simulink model "control_cdr_hybrid"  (Simulink 7.8)
settings: Solver=ode5  StartTime=0.0  StopTime=100  FixedStep=0.001  RelTol=1e-3
undefined symbols (not defined in the file): DamperOFF, DiscIntNeverNeededParam, Ki_L1, Ki_R1, Ki_R3, Kp_L1, Kp_R1, Kp_R2, Kp_R3, Matlab_version, Output_File, Output_file_n, Plant_inputs_num, Plant_outputs_num, polys, RecurDyn, RecurDyn_controltimestep, RecurDyn_model, RecurDyn_model_n, sigbuilder_block, SpringOFF, StaticTorque_RW1, StaticTorque_RW2, Ts, Tuning, Wheel_Vel
(part 1 of 2)
settings Model: Creator=sonyi  LastModifiedBy=ecsl
settings OptimizationCC: InitFltsAndDblsToZero=on
settings DebuggingCC: FcnCallInpInsideContextMsg=Use local settings  StrictBusMsg=Warning
settings SimEventsCC: propDiagStatOutput=1

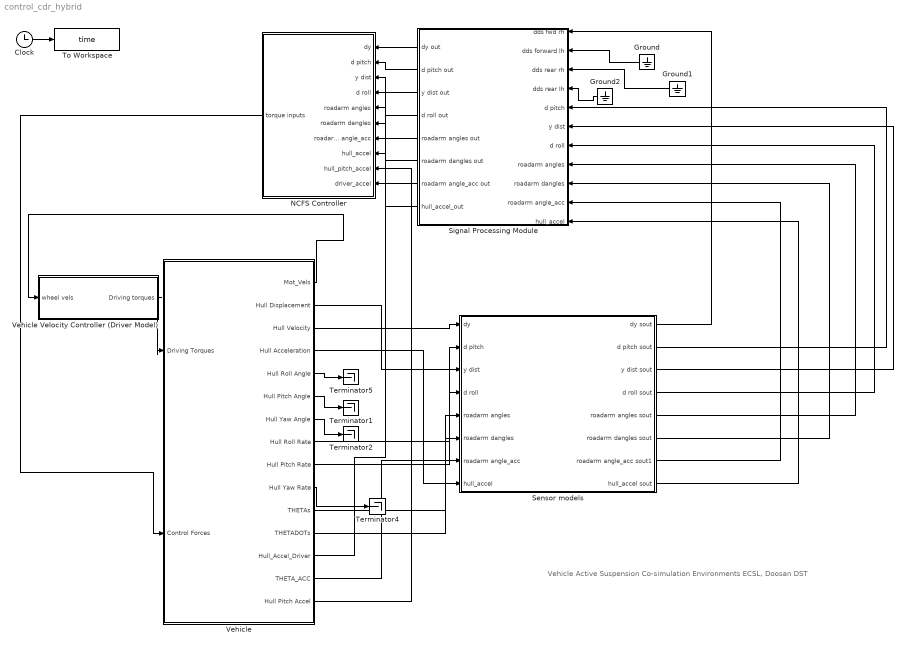
== system control_cdr_hybrid ==
  note: Vehicle Active Suspension Co-simulation Environments
      | ECSL, Doosan DST
  Clock : Clock
  Ground : Ground
  Ground1 : Ground
  Ground2 : Ground
  NCFS Controller : Subsystem
  Sensor models : Subsystem
  Signal Processing Module : Subsystem
  Terminator{1..2,4..5} (4 alike) : Terminator
  To Workspace : ToWorkspace  VariableName=time  SampleTime=-1  SaveFormat=Array
  Vehicle : Subsystem
  Vehicle Velocity Controller (Driver Model) : Subsystem
  wires:
  Vehicle/1(Mot_Vels) -> Vehicle Velocity Controller (Driver Model)/1(wheel vels)
  Clock/1 -> To Workspace/1
  Signal Processing Module/1(dy out) -> NCFS Controller/1(dy)
  Signal Processing Module/3(y dist out) -> NCFS Controller/3(y dist)
  Signal Processing Module/2(d pitch out) -> NCFS Controller/2(d pitch)
  Signal Processing Module/5(roadarm angles out) -> NCFS Controller/5(roadarm angles)
  Signal Processing Module/4(d roll out) -> NCFS Controller/4(d roll)
  Signal Processing Module/6(roadarm dangles out) -> NCFS Controller/6(roadarm dangles)
  Sensor models/1(dy sout) -> Signal Processing Module/1(dds fwd rh)
  Sensor models/2(d pitch sout) -> Signal Processing Module/5(d pitch)
  Sensor models/3(y dist sout) -> Signal Processing Module/6(y dist)
  Sensor models/4(d roll sout) -> Signal Processing Module/7(d roll)
  Sensor models/5(roadarm angles sout) -> Signal Processing Module/8(roadarm angles)
  Sensor models/6(roadarm dangles sout) -> Signal Processing Module/9(roadarm dangles)
  NCFS Controller/1(torque inputs) -> Vehicle/2(Control Forces)
  Sensor models/7(roadarm angle_acc sout1) -> Signal Processing Module/10(roadarm angle_acc)
  Signal Processing Module/7(roadarm angle_acc out) -> NCFS Controller/7(roadarm angle_acc)
  Sensor models/8(hull_accel sout) -> Signal Processing Module/11(hull_accel)
  Signal Processing Module/8(hull_accel_out) -> NCFS Controller/8(hull_accel)
  Ground/1 -> Signal Processing Module/2(dds forward lh)
  Ground1/1 -> Signal Processing Module/3(dds rear rh)
  Ground2/1 -> Signal Processing Module/4(dds rear lh)
  Vehicle/2(Hull Displacement) -> Sensor models/3(y dist)
  Vehicle/3(Hull Velocity) -> Sensor models/1(dy)
  Vehicle/4(Hull Acceleration) -> Sensor models/8(hull_accel)
  Vehicle/8(Hull Roll Rate) -> Sensor models/4(d roll)
  Vehicle/11(THETAs) -> Sensor models/5(roadarm angles)
  Vehicle/12(THETADOTs) -> Sensor models/6(roadarm dangles)
  Vehicle/5(Hull Roll Angle) -> Terminator5/1
  Vehicle/6(Hull Pitch Angle) -> Terminator1/1
  Vehicle/7(Hull Yaw Angle) -> Terminator2/1
  Vehicle/9(Hull Pitch Rate) -> Sensor models/2(d pitch)
  Vehicle/10(Hull Yaw Rate) -> Terminator4/1
  Vehicle/14(THETA_ACC) -> Sensor models/7(roadarm angle_acc)
  Vehicle Velocity Controller (Driver Model)/1(Driving torques) -> Vehicle/1(Driving Torques)
  Vehicle/15(Hull Pitch Accel) -> NCFS Controller/9(hull_pitch_accel)
  Vehicle/13(Hull_Accel_Driver) -> NCFS Controller/10(driver_accel)

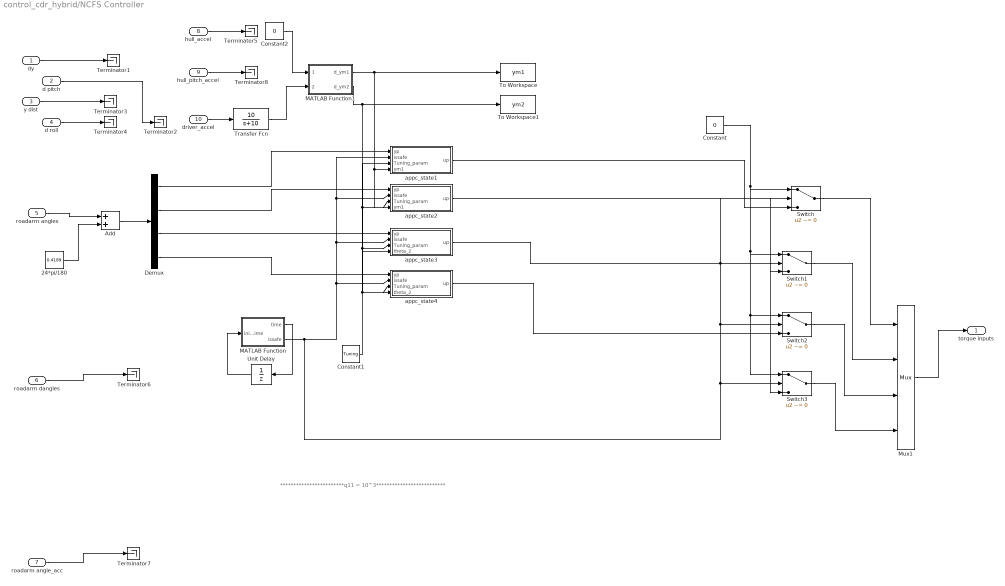
== system control_cdr_hybrid/NCFS Controller ==
  note: ************************q11 = 10^3**************************
  dy : Inport
  d pitch : Inport  Port=2
  y dist : Inport  Port=3
  d roll : Inport  Port=4
  roadarm angles : Inport  Port=5
  roadarm dangles : Inport  Port=6
  roadarm angle_acc : Inport  Port=7
  hull_accel : Inport  Port=8
  hull_pitch_accel : Inport  Port=9
  driver_accel : Inport  Port=10
  24*pi/180 : Constant  Value=0.4189
  Add : Sum
  Constant : Constant  Value=0
  Constant1 : Constant  Value=Tuning
  Constant2 : Constant  Value=0
  Demux : Demux
  MATLAB Function : MATLAB Function  TreatAsAtomicUnit=on
  MATLAB Function1 : MATLAB Function  TreatAsAtomicUnit=on
  Mux1 : Mux
  Switch{,1..3} (4 alike) : Switch  Criteria=u2 ~= 0
  Terminator{1..8} (8 alike) : Terminator
  To Workspace : ToWorkspace  VariableName=ym1  SampleTime=-1  SaveFormat=Array
  To Workspace1 : ToWorkspace  VariableName=ym2  SampleTime=-1  SaveFormat=Array
  Transfer Fcn : TransferFcn  Numerator=[10]  Denominator=[1 10]
  Unit Delay : UnitDelay  X0=3000  SampleTime=-1
  appc_state1 : Subsystem
  appc_state2 : Subsystem
  appc_state3 : Subsystem
  appc_state4 : Subsystem
  torque inputs : Outport
  wires:
  dy/1 -> Terminator1/1
  y dist/1 -> Terminator3/1
  d roll/1 -> Terminator4/1
  Mux1/1 -> torque inputs/1
  roadarm angles/1 -> Add/1
  24*pi/180/1 -> Add/2
  Add/1 -> Demux/1
  d pitch/1 -> Terminator2/1
  roadarm dangles/1 -> Terminator6/1
  roadarm angle_acc/1 -> Terminator7/1
  Demux/1 -> appc_state1/1(yp)
  Demux/2 -> appc_state2/1(yp)
  Demux/3 -> appc_state3/1(yp)
  Demux/4 -> appc_state4/1(yp)
  Constant1/1 -> appc_state1/3(Tuning_param), appc_state2/3(Tuning_param), appc_state3/3(Tuning_param), appc_state4/3(Tuning_param)
  appc_state3/1(up) -> Switch2/3
  appc_state4/1(up) -> Switch3/3
  appc_state1/1(up) -> Switch/3
  Constant/1 -> Switch/1, Switch3/1, Switch2/1, Switch1/1
  Unit Delay/1 -> MATLAB Function/1(init_time)
  MATLAB Function/1(time) -> Unit Delay/1
  MATLAB Function/2(issafe) -> appc_state4/2(issafe), appc_state3/2(issafe), appc_state2/2(issafe), appc_state1/2(issafe), Switch/2, Switch1/2, Switch2/2, Switch3/2
  appc_state2/1(up) -> Switch1/3
  MATLAB Function1/1(d_ym1) -> To Workspace/1, appc_state1/4(ym1), appc_state2/4(ym1)
  MATLAB Function1/2(d_ym2) -> To Workspace1/1, appc_state3/4(theta_2), appc_state4/4(theta_2)
  Switch/1 -> Mux1/1
  Switch1/1 -> Mux1/2
  Switch2/1 -> Mux1/3
  Switch3/1 -> Mux1/4
  Constant2/1 -> MATLAB Function1/1(pitch_acc)
  Transfer Fcn/1 -> MATLAB Function1/2(hull_acc)
  hull_pitch_accel/1 -> Terminator8/1
  hull_accel/1 -> Terminator5/1
  driver_accel/1 -> Transfer Fcn/1

== system control_cdr_hybrid/Sensor models ==
  dy : Inport
  d pitch : Inport  Port=2
  y dist : Inport  Port=3
  d roll : Inport  Port=4
  roadarm angles : Inport  Port=5
  roadarm dangles : Inport  Port=6
  roadarm angle_acc : Inport  Port=7
  hull_accel : Inport  Port=8
  dy sout : Outport
  d pitch sout : Outport  Port=2
  y dist sout : Outport  Port=3
  d roll sout : Outport  Port=4
  roadarm angles sout : Outport  Port=5
  roadarm dangles sout : Outport  Port=6
  roadarm angle_acc sout1 : Outport  Port=7
  hull_accel sout : Outport  Port=8
  wires:
  dy/1 -> dy sout/1
  y dist/1 -> y dist sout/1
  d pitch/1 -> d pitch sout/1
  roadarm angles/1 -> roadarm angles sout/1
  d roll/1 -> d roll sout/1
  roadarm dangles/1 -> roadarm dangles sout/1
  roadarm angle_acc/1 -> roadarm angle_acc sout1/1
  hull_accel/1 -> hull_accel sout/1

== system control_cdr_hybrid/Signal Processing Module ==
  dds fwd rh : Inport
  dds forward lh : Inport  Port=2
  dds rear rh : Inport  Port=3
  dds rear lh : Inport  Port=4
  d pitch : Inport  Port=5
  y dist : Inport  Port=6
  d roll : Inport  Port=7
  roadarm angles : Inport  Port=8
  roadarm dangles : Inport  Port=9
  roadarm angle_acc : Inport  Port=10
  hull_accel : Inport  Port=11
  Terminator : Terminator
  Terminator1 : Terminator
  Terminator2 : Terminator
  dy out : Outport
  d pitch out : Outport  Port=2
  y dist out : Outport  Port=3
  d roll out : Outport  Port=4
  roadarm angles out : Outport  Port=5
  roadarm dangles out : Outport  Port=6
  roadarm angle_acc out : Outport  Port=7
  hull_accel_out : Outport  Port=8
  wires:
  dds fwd rh/1 -> dy out/1
  y dist/1 -> y dist out/1
  d pitch/1 -> d pitch out/1
  roadarm angles/1 -> roadarm angles out/1
  d roll/1 -> d roll out/1
  roadarm dangles/1 -> roadarm dangles out/1
  roadarm angle_acc/1 -> roadarm angle_acc out/1
  hull_accel/1 -> hull_accel_out/1
  dds rear lh/1 -> Terminator2/1
  dds rear rh/1 -> Terminator1/1
  dds forward lh/1 -> Terminator/1

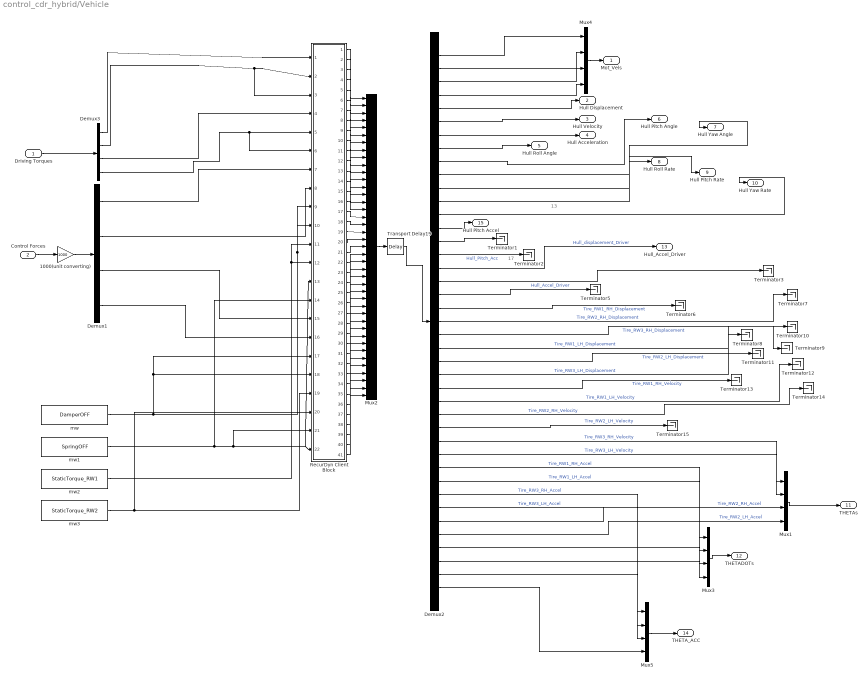
== system control_cdr_hybrid/Vehicle ==
  note: 13
  note: 17
  Driving Torques : Inport
  Control Forces : Inport  Port=2
  1000(unit converting) : Gain  Gain=1000
  Demux1 : Demux
  Demux2 : Demux  Outputs=41
  Demux3 : Demux
  Mux{1,3..5} (4 alike) : Mux
  Mux2 : Mux  Inputs=41
  RecurDyn Client Block : Subsystem
      mask Display: image(imread('basic_recurdyn2_client.TIF'))
  Terminator{1..3,5..15} (14 alike) : Terminator
  Transport Delay19 : TransportDelay  DelayTime=0.001
  mw : Constant  Value=DamperOFF
  mw1 : Constant  Value=SpringOFF
  mw2 : Constant  Value=StaticTorque_RW1
  mw3 : Constant  Value=StaticTorque_RW2
  Mot_Vels : Outport
  Hull Displacement : Outport  Port=2
  Hull Velocity : Outport  Port=3
  Hull Acceleration : Outport  Port=4
  Hull Roll Angle : Outport  Port=5
  Hull Pitch Angle : Outport  Port=6
  Hull Yaw Angle : Outport  Port=7
  Hull Roll Rate : Outport  Port=8
  Hull Pitch Rate : Outport  Port=9
  Hull Yaw Rate : Outport  Port=10
  THETAs : Outport  Port=11
  THETADOTs : Outport  Port=12
  Hull_Accel_Driver : Outport  Port=13
  THETA_ACC : Outport  Port=14
  Hull Pitch Accel : Outport  Port=15
  wires:
  Demux3/2 -> RecurDyn Client Block/2("Mot_Input_R2            "), RecurDyn Client Block/3("Mot_Input_R3            ")
  Demux3/1 -> RecurDyn Client Block/1("Mot_Input_R1            ")
  Transport Delay19/1 -> Demux2/1
  Mux2/1 -> Transport Delay19/1
  Driving Torques/1 -> Demux3/1
  Control Forces/1 -> 1000(unit converting)/1
  1000(unit converting)/1 -> Demux1/1
  Demux1/1 -> RecurDyn Client Block/7("Torque_RW1_RH@Arm1      ")
  Demux1/2 -> RecurDyn Client Block/8("Torque_RW1_LH@Arm1      ")
  mw/1 -> RecurDyn Client Block/9("DamperOFF_RW1_RH@Arm1   "), RecurDyn Client Block/10("DamperOFF_RW1_LH@Arm1   "), RecurDyn Client Block/17("DamperOFF_RW2_RH@Arm2   "), RecurDyn Client Block/18("DamperOFF_RW2_LH@Arm2   ")
  mw2/1 -> RecurDyn Client Block/11(StaticTorque_RW1_RH@Arm1), RecurDyn Client Block/12(StaticTorque_RW1_LH@Arm1)
  mw1/1 -> RecurDyn Client Block/13("SpringOFF_RW1_RH@Arm1   "), RecurDyn Client Block/21("SpringOFF_RW2_RH@Arm2   "), RecurDyn Client Block/22("SpringOFF_RW2_LH@Arm2   "), RecurDyn Client Block/14("SpringOFF_RW1_LH@Arm1   ")
  Demux1/3 -> RecurDyn Client Block/15("Torque_RW2_RH@Arm2      ")
  Demux1/4 -> RecurDyn Client Block/16("Torque_RW2_LH@Arm2      ")
  Mux4/1 -> Mot_Vels/1
  Demux2/1 -> Mux4/1
  Demux2/2 -> Mux4/2
  Demux2/3 -> Mux4/3
  Demux2/4 -> Mux4/4
  Demux2/5 -> Hull Displacement/1
  Demux2/6 -> Hull Velocity/1
  Demux2/7 -> Hull Acceleration/1
  Demux2/8 -> Hull Roll Angle/1
  Demux2/9 -> Hull Pitch Angle/1
  Demux2/10 -> Hull Yaw Angle/1
  Demux2/11 -> Hull Roll Rate/1
  Demux2/12 -> Hull Pitch Rate/1
  Demux2/13 -> Hull Yaw Rate/1
  Mux3/1 -> THETADOTs/1
  Mux1/1 -> THETAs/1
  Mux5/1 -> THETA_ACC/1
  Demux2/14 -> Hull Pitch Accel/1
  Demux2/15 -> Terminator1/1
  Demux2/16 -> Terminator2/1  "Hull_Pitch_Acc"
  Demux2/17 -> Hull_Accel_Driver/1  "Hull_displacement_Driver"
  Demux2/18 -> Terminator3/1
  Demux2/19 -> Terminator5/1  "Hull_Accel_Driver"
  Demux2/41 -> Mux5/4
  Demux2/40 -> Mux5/3
  Demux2/39 -> Mux3/4
  Demux2/38 -> Mux3/3
  Demux2/37 -> Mux1/4  "Tire_RW2_LH_Accel"
  Demux2/36 -> Mux1/3  "Tire_RW2_RH_Accel"
  Demux2/35 -> Mux5/2  "Tire_RW3_LH_Accel"
  Demux2/34 -> Mux5/1  "Tire_RW3_RH_Accel"
  Demux2/33 -> Mux3/2  "Tire_RW1_LH_Accel"
  Demux2/32 -> Mux3/1  "Tire_RW1_RH_Accel"
  Demux2/31 -> Mux1/2  "Tire_RW3_LH_Velocity"
  Demux2/30 -> Mux1/1  "Tire_RW3_RH_Velocity"
  Demux2/20 -> Terminator6/1  "Tire_RW1_RH_Displacement"
  Demux2/21 -> Terminator7/1  "Tire_RW2_RH_Displacement"
  Demux2/22 -> Terminator10/1  "Tire_RW3_RH_Displacement"
  Demux2/23 -> Terminator8/1  "Tire_RW1_LH_Displacement"
  Demux2/24 -> Terminator11/1  "Tire_RW2_LH_Displacement"
  Demux2/25 -> Terminator9/1  "Tire_RW3_LH_Displacement"
  Demux2/26 -> Terminator13/1  "Tire_RW1_RH_Velocity"
  Demux2/27 -> Terminator12/1  "Tire_RW1_LH_Velocity"
  Demux2/28 -> Terminator14/1  "Tire_RW2_RH_Velocity"
  Demux2/29 -> Terminator15/1  "Tire_RW2_LH_Velocity"
  RecurDyn Client Block/1("Mot_R1_Encoder_Output   ") -> Mux2/1
  RecurDyn Client Block/2("Mot_R2_Encoder_Output   ") -> Mux2/2
  RecurDyn Client Block/3("Mot_L1_Encoder_Output   ") -> Mux2/3
  RecurDyn Client Block/4("Mot_L2_Encoder_Output   ") -> Mux2/4
  RecurDyn Client Block/5("Hull_Displacement       ") -> Mux2/5
  RecurDyn Client Block/6("Hull_Velocity           ") -> Mux2/6
  RecurDyn Client Block/7("Hull_Accel              ") -> Mux2/7
  RecurDyn Client Block/8("Hull_Roll               ") -> Mux2/8
  RecurDyn Client Block/9("Hull_Pitch              ") -> Mux2/9
  RecurDyn Client Block/10("Hull_Yaw                ") -> Mux2/10
  RecurDyn Client Block/11("Hull_RollRate           ") -> Mux2/11
  RecurDyn Client Block/12("Hull_PitchRate          ") -> Mux2/12
  RecurDyn Client Block/13("Hull_YawRate            ") -> Mux2/13
  RecurDyn Client Block/14("Hull_PitchAcc           ") -> Mux2/14
  RecurDyn Client Block/15(Hull_Displacement_Driver) -> Mux2/15
  RecurDyn Client Block/16("Hull_Velocity_Driver    ") -> Mux2/16
  RecurDyn Client Block/17("Hull_Accel_Driver       ") -> Mux2/17
  RecurDyn Client Block/18(Tire_RW1_RH_Displacement) -> Mux2/18
  RecurDyn Client Block/19(Tire_RW2_RH_Displacement) -> Mux2/19
  RecurDyn Client Block/20(Tire_RW1_LH_Displacement) -> Mux2/20
  RecurDyn Client Block/21(Tire_RW2_LH_Displacement) -> Mux2/21
  RecurDyn Client Block/22("Tire_RW1_RH_Velocity    ") -> Mux2/22
  RecurDyn Client Block/23("Tire_RW1_LH_Velocity    ") -> Mux2/23
  RecurDyn Client Block/24("Tire_RW2_RH_Velocity    ") -> Mux2/24
  RecurDyn Client Block/25("Tire_RW2_LH_Velocity    ") -> Mux2/25
  RecurDyn Client Block/26("Tire_RW1_RH_Accel       ") -> Mux2/26
  RecurDyn Client Block/27("Tire_RW1_LH_Accel       ") -> Mux2/27
  RecurDyn Client Block/28("Tire_RW2_RH_Accel       ") -> Mux2/28
  RecurDyn Client Block/29("Tire_RW2_LH_Accel       ") -> Mux2/29
  RecurDyn Client Block/30("Theta_RW1_RH@Arm1       ") -> Mux2/30
  RecurDyn Client Block/31("Theta_RW1_LH@Arm1       ") -> Mux2/31
  RecurDyn Client Block/32("Thetadot_RW1_RH@Arm1    ") -> Mux2/32
  RecurDyn Client Block/33("Thetadot_RW1_LH@Arm1    ") -> Mux2/33
  RecurDyn Client Block/34("Theta_Accel_RW1_RH@Arm1 ") -> Mux2/34
  RecurDyn Client Block/35("Theta_Accel_RW1_LH@Arm1 ") -> Mux2/35
  RecurDyn Client Block/36("Theta_RW2_RH@Arm2       ") -> Mux2/36
  RecurDyn Client Block/37("Theta_RW2_LH@Arm2       ") -> Mux2/37
  RecurDyn Client Block/38("Thetadot_RW2_RH@Arm2    ") -> Mux2/38
  RecurDyn Client Block/39("Thetadot_RW2_LH@Arm2    ") -> Mux2/39
  RecurDyn Client Block/40("Theta_Accel_RW2_RH@Arm2 ") -> Mux2/40
  RecurDyn Client Block/41("Theta_Accel_RW2_LH@Arm2 ") -> Mux2/41
  Demux3/3 -> RecurDyn Client Block/4("Mot_Input_L1            ")
  Demux3/4 -> RecurDyn Client Block/5("Mot_Input_L2            "), RecurDyn Client Block/6("Mot_Input_L3            ")
  mw3/1 -> RecurDyn Client Block/19(StaticTorque_RW2_RH@Arm2), RecurDyn Client Block/20(StaticTorque_RW2_LH@Arm2)

== system control_cdr_hybrid/Vehicle Velocity Controller (Driver Model) ==
  wheel vels : Inport
  Demux1 : Demux
  Gain : Gain  Gain=Wheel_Vel
  Gain1 : Gain
  L1_controller : Subsystem
  Mux2 : Mux
  R1_controller : Subsystem
  R2_controller : Subsystem
  R3_controller : Subsystem
  normal case velocity control profile : Subsystem  Tag=STV Subsys  LoadFcn=sigbuilder_block('load');  StartFcn=sigbuilder_block('start');  StopFcn=sigbuilder_block('stop');  ClipboardFcn=sigbuilder_block('clipboard');  mask(Sigbuilder block){}
      mask help: Sigbuilder GUI
      mask init:
      | if ~strcmp(get_param(bdroot(gcbh),'SimulationStatus'),'stopped') tuvar = sigbuilder_block('maskInit'); end
      settings: CopyFcn=sigbuilder_block('copy');  DeleteFcn=sigbuilder_block('delete');  ModelCloseFcn=sigbuilder_block('modelClose');  PreSaveFcn=sigbuilder_block('preSave');  NameChangeFcn=sigbuilder_block('namechange');  OpenFcn=sigbuilder_block('open',[75.75 124.5 830.25 492 ]);  CloseFcn=sigbuilder_block('close');
      mask Display: plot(0,0,100,100,[10,10,40,40,10],[80,20,20,80,80],[40,10],[50,50], [40,27,10],[65,72,56],[40,25,25,10],[28,28,43,43]);
  Driving torques : Outport
  tag scope: Vehicle_Velocity=global
  wires:
  R1_controller/1(Torque_R1) -> Mux2/1
  Demux1/1 -> R1_controller/2(Feedback_Vel)
  R2_controller/1(Torque_R2) -> Mux2/2
  Demux1/2 -> R2_controller/2(Feedback_Vel)
  R3_controller/1(Torque_R3) -> Mux2/3
  Demux1/3 -> R3_controller/2(Feedback_Vel)
  L1_controller/1(Torque_L1) -> Mux2/4
  Demux1/4 -> L1_controller/2(Feedback_Vel)
  Gain/1 -> R1_controller/1(Ref_Vel), R2_controller/1(Ref_Vel), R3_controller/1(Ref_Vel), L1_controller/1(Ref_Vel)
  Mux2/1 -> Driving torques/1
  wheel vels/1 -> Gain1/1
  Gain1/1 -> Demux1/1
  normal case velocity control profile/1(Signal 1) -> Gain/1, [Vehicle_Velocity]

== system control_cdr_hybrid/NCFS Controller/appc_state1 ==
  yp : Inport
  issafe : Inport  Port=2
  Tuning_param : Inport  Port=3
  ym1 : Inport  Port=4
  -3,-4,-5 : Constant  Value=polys
  Add1 : Sum
  Constant1 : Constant  Value=[-0.0140; -0.0440; 0.0013; 113.8736]
  Constant2 : Constant  Value=0.3
  adaptive_interface_con : Subsystem
  online estimator : Subsystem
  up : Outport
  wires:
  adaptive_interface_con/1(up) -> up/1, online estimator/1(u)
  yp/1 -> online estimator/2(y), adaptive_interface_con/1(yp)
  Tuning_param/1 -> online estimator/3(Tuning_param)
  Constant1/1 -> online estimator/4(param_initialcondition)
  -3,-4,-5/1 -> adaptive_interface_con/4(eig-poly)
  issafe/1 -> online estimator/5(issafe)
  online estimator/1(estimated_param) -> adaptive_interface_con/2(plant_param)
  Constant2/1 -> Add1/1
  Add1/1 -> adaptive_interface_con/3(ym)
  ym1/1 -> Add1/2

== system control_cdr_hybrid/NCFS Controller/appc_state2 ==
  yp : Inport
  issafe : Inport  Port=2
  Tuning_param : Inport  Port=3
  ym1 : Inport  Port=4
  -3,-4,-5 : Constant  Value=polys
  Add1 : Sum
  Constant1 : Constant  Value=[-0.0140; -0.0440; 0.0013; 113.8736]
  Constant3 : Constant  Value=0.3
  adaptive_interface_con1 : Subsystem
  online estimator : Subsystem
  up : Outport
  wires:
  adaptive_interface_con1/1(up) -> up/1, online estimator/1(u)
  yp/1 -> online estimator/2(y), adaptive_interface_con1/1(yp)
  Tuning_param/1 -> online estimator/3(Tuning_param)
  Constant1/1 -> online estimator/4(param_initialcondition)
  Add1/1 -> adaptive_interface_con1/3(ym)
  -3,-4,-5/1 -> adaptive_interface_con1/4(eig-poly)
  issafe/1 -> online estimator/5(issafe)
  online estimator/1(estimated_param) -> adaptive_interface_con1/2(plant_param)
  Constant3/1 -> Add1/1
  ym1/1 -> Add1/2

== system control_cdr_hybrid/NCFS Controller/appc_state3 ==
  yp : Inport
  issafe : Inport  Port=2
  Tuning_param : Inport  Port=3
  theta_2 : Inport  Port=4
  -3,-4,-5 : Constant  Value=polys
  Add : Sum
  Constant : Constant  Value=0.4189
  Constant1 : Constant  Value=[0.0037; -0.0410; 0.0013; 113.8736]
  adaptive_interface_con : Subsystem
  online estimator : Subsystem
  up : Outport
  wires:
  adaptive_interface_con/1(up) -> up/1, online estimator/1(u)
  yp/1 -> online estimator/2(y), adaptive_interface_con/1(yp)
  Tuning_param/1 -> online estimator/3(Tuning_param)
  Constant1/1 -> online estimator/4(param_initialcondition)
  -3,-4,-5/1 -> adaptive_interface_con/4(eig-poly)
  issafe/1 -> online estimator/5(issafe)
  online estimator/1(estimated_param) -> adaptive_interface_con/2(plant_param)
  theta_2/1 -> Add/1
  Add/1 -> adaptive_interface_con/3(ym)
  Constant/1 -> Add/2

== system control_cdr_hybrid/NCFS Controller/appc_state4 ==
  yp : Inport
  issafe : Inport  Port=2
  Tuning_param : Inport  Port=3
  theta_2 : Inport  Port=4
  -3,-4,-5 : Constant  Value=polys
  Add : Sum
  Constant : Constant  Value=0.4189
  Constant1 : Constant  Value=[0.0037; -0.0410; 0.0013; 113.8736]
  adaptive_interface_con : Subsystem
  online estimator : Subsystem
  up : Outport
  wires:
  adaptive_interface_con/1(up) -> up/1, online estimator/1(u)
  yp/1 -> online estimator/2(y), adaptive_interface_con/1(yp)
  Tuning_param/1 -> online estimator/3(Tuning_param)
  Constant1/1 -> online estimator/4(param_initialcondition)
  -3,-4,-5/1 -> adaptive_interface_con/4(eig-poly)
  issafe/1 -> online estimator/5(issafe)
  online estimator/1(estimated_param) -> adaptive_interface_con/2(plant_param)
  theta_2/1 -> Add/1
  Add/1 -> adaptive_interface_con/3(ym)
  Constant/1 -> Add/2

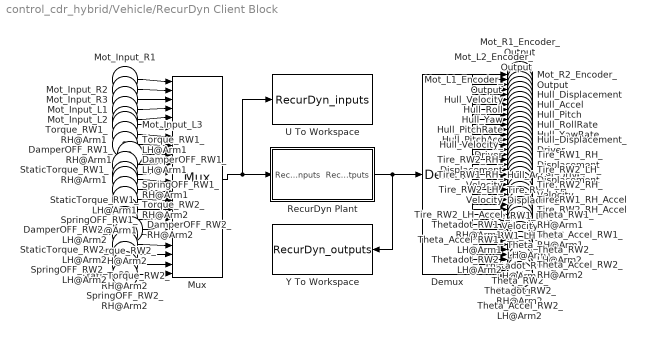
== system control_cdr_hybrid/Vehicle/RecurDyn Client Block ==
  "Mot_Input_R1            " : Inport
  "Mot_Input_R2            " : Inport  Port=2
  "Mot_Input_R3            " : Inport  Port=3
  "Mot_Input_L1            " : Inport  Port=4
  "Mot_Input_L2            " : Inport  Port=5
  "Mot_Input_L3            " : Inport  Port=6
  "Torque_RW1_RH@Arm1      " : Inport  Port=7
  "Torque_RW1_LH@Arm1      " : Inport  Port=8
  "DamperOFF_RW1_RH@Arm1   " : Inport  Port=9
  "DamperOFF_RW1_LH@Arm1   " : Inport  Port=10
  StaticTorque_RW1_RH@Arm1 : Inport  Port=11
  StaticTorque_RW1_LH@Arm1 : Inport  Port=12
  "SpringOFF_RW1_RH@Arm1   " : Inport  Port=13
  "SpringOFF_RW1_LH@Arm1   " : Inport  Port=14
  "Torque_RW2_RH@Arm2      " : Inport  Port=15
  "Torque_RW2_LH@Arm2      " : Inport  Port=16
  "DamperOFF_RW2_RH@Arm2   " : Inport  Port=17
  "DamperOFF_RW2_LH@Arm2   " : Inport  Port=18
  StaticTorque_RW2_RH@Arm2 : Inport  Port=19
  StaticTorque_RW2_LH@Arm2 : Inport  Port=20
  "SpringOFF_RW2_RH@Arm2   " : Inport  Port=21
  "SpringOFF_RW2_LH@Arm2   " : Inport  Port=22
  Demux : Demux  Outputs=41
  Mux : Mux  Inputs=22
  RecurDyn Plant : Subsystem  mask(Recurdyn/Plant){RecurDyn_model_name=RecurDyn_model, Output_File_Name_=Output_File, RecurDyn_=RecurDyn, Matlab_version_=Matlab_version, RecurDyn_controltimestep_=RecurDyn_controltimestep, RecurDyn_step_=100, Waitingtime=1000, RecurDyn_static_=off, RecurDyn_show_=on, RecurDyn_ani_=on, Create_Output_Folder_=off}
      mask prompts: Output_File_Name_ "Output File Name"; RecurDyn_ "RecurDyn_install_directory"; Matlab_version_ "Matlab version"; RecurDyn_controltimestep_ "Sampling period"; RecurDyn_step_ "RecurDyn_step"; Waitingtime "Waiting time"; RecurDyn_static_ "Static analysis"; RecurDyn_show_ "RecurDyn_show"; RecurDyn_ani_ "RecurDyn_animation"; Create_Output_Folder_ "Create Output Folder"
      mask help:
      | Simulate any Recurdyn Dynamics Model in Recurdyn/Solver
      | Plant inputs and Plant outputs are transfered every sampling time
      | Here, sampling time is determined by sampling period (Control time step)
      mask Display: disp( 'Dynamic Model' )
  U To Workspace : ToWorkspace  VariableName=RecurDyn_inputs  SaveFormat=Array
  Y To Workspace : ToWorkspace  VariableName=RecurDyn_outputs  SaveFormat=Array
  "Mot_R1_Encoder_Output   " : Outport
  "Mot_R2_Encoder_Output   " : Outport  Port=2
  "Mot_L1_Encoder_Output   " : Outport  Port=3
  "Mot_L2_Encoder_Output   " : Outport  Port=4
  "Hull_Displacement       " : Outport  Port=5
  "Hull_Velocity           " : Outport  Port=6
  "Hull_Accel              " : Outport  Port=7
  "Hull_Roll               " : Outport  Port=8
  "Hull_Pitch              " : Outport  Port=9
  "Hull_Yaw                " : Outport  Port=10
  "Hull_RollRate           " : Outport  Port=11
  "Hull_PitchRate          " : Outport  Port=12
  "Hull_YawRate            " : Outport  Port=13
  "Hull_PitchAcc           " : Outport  Port=14
  Hull_Displacement_Driver : Outport  Port=15
  "Hull_Velocity_Driver    " : Outport  Port=16
  "Hull_Accel_Driver       " : Outport  Port=17
  Tire_RW1_RH_Displacement : Outport  Port=18
  Tire_RW2_RH_Displacement : Outport  Port=19
  Tire_RW1_LH_Displacement : Outport  Port=20
  Tire_RW2_LH_Displacement : Outport  Port=21
  "Tire_RW1_RH_Velocity    " : Outport  Port=22
  "Tire_RW1_LH_Velocity    " : Outport  Port=23
  "Tire_RW2_RH_Velocity    " : Outport  Port=24
  "Tire_RW2_LH_Velocity    " : Outport  Port=25
  "Tire_RW1_RH_Accel       " : Outport  Port=26
  "Tire_RW1_LH_Accel       " : Outport  Port=27
  "Tire_RW2_RH_Accel       " : Outport  Port=28
  "Tire_RW2_LH_Accel       " : Outport  Port=29
  "Theta_RW1_RH@Arm1       " : Outport  Port=30
  "Theta_RW1_LH@Arm1       " : Outport  Port=31
  "Thetadot_RW1_RH@Arm1    " : Outport  Port=32
  "Thetadot_RW1_LH@Arm1    " : Outport  Port=33
  "Theta_Accel_RW1_RH@Arm1 " : Outport  Port=34
  "Theta_Accel_RW1_LH@Arm1 " : Outport  Port=35
  "Theta_RW2_RH@Arm2       " : Outport  Port=36
  "Theta_RW2_LH@Arm2       " : Outport  Port=37
  "Thetadot_RW2_RH@Arm2    " : Outport  Port=38
  "Thetadot_RW2_LH@Arm2    " : Outport  Port=39
  "Theta_Accel_RW2_RH@Arm2 " : Outport  Port=40
  "Theta_Accel_RW2_LH@Arm2 " : Outport  Port=41
  wires:
  RecurDyn Plant/1(RecurDyn_outputs) -> Demux/1, Y To Workspace/1
  Mux/1 -> RecurDyn Plant/1(" RecurDyn_inputs"), U To Workspace/1
  Demux/1 -> "Mot_R1_Encoder_Output   "/1
  Demux/2 -> "Mot_R2_Encoder_Output   "/1
  Demux/3 -> "Mot_L1_Encoder_Output   "/1
  Demux/4 -> "Mot_L2_Encoder_Output   "/1
  Demux/5 -> "Hull_Displacement       "/1
  Demux/6 -> "Hull_Velocity           "/1
  Demux/7 -> "Hull_Accel              "/1
  Demux/8 -> "Hull_Roll               "/1
  Demux/9 -> "Hull_Pitch              "/1
  Demux/10 -> "Hull_Yaw                "/1
  Demux/11 -> "Hull_RollRate           "/1
  Demux/12 -> "Hull_PitchRate          "/1
  Demux/13 -> "Hull_YawRate            "/1
  Demux/14 -> "Hull_PitchAcc           "/1
  Demux/15 -> Hull_Displacement_Driver/1
  Demux/16 -> "Hull_Velocity_Driver    "/1
  Demux/17 -> "Hull_Accel_Driver       "/1
  Demux/18 -> Tire_RW1_RH_Displacement/1
  Demux/19 -> Tire_RW2_RH_Displacement/1
  Demux/20 -> Tire_RW1_LH_Displacement/1
  Demux/21 -> Tire_RW2_LH_Displacement/1
  Demux/22 -> "Tire_RW1_RH_Velocity    "/1
  Demux/23 -> "Tire_RW1_LH_Velocity    "/1
  Demux/24 -> "Tire_RW2_RH_Velocity    "/1
  Demux/25 -> "Tire_RW2_LH_Velocity    "/1
  Demux/26 -> "Tire_RW1_RH_Accel       "/1
  Demux/27 -> "Tire_RW1_LH_Accel       "/1
  Demux/28 -> "Tire_RW2_RH_Accel       "/1
  Demux/29 -> "Tire_RW2_LH_Accel       "/1
  Demux/30 -> "Theta_RW1_RH@Arm1       "/1
  Demux/31 -> "Theta_RW1_LH@Arm1       "/1
  Demux/32 -> "Thetadot_RW1_RH@Arm1    "/1
  Demux/33 -> "Thetadot_RW1_LH@Arm1    "/1
  Demux/34 -> "Theta_Accel_RW1_RH@Arm1 "/1
  Demux/35 -> "Theta_Accel_RW1_LH@Arm1 "/1
  Demux/36 -> "Theta_RW2_RH@Arm2       "/1
  Demux/37 -> "Theta_RW2_LH@Arm2       "/1
  Demux/38 -> "Thetadot_RW2_RH@Arm2    "/1
  Demux/39 -> "Thetadot_RW2_LH@Arm2    "/1
  Demux/40 -> "Theta_Accel_RW2_RH@Arm2 "/1
  Demux/41 -> "Theta_Accel_RW2_LH@Arm2 "/1
  "Mot_Input_R1            "/1 -> Mux/1
  "Mot_Input_R2            "/1 -> Mux/2
  "Mot_Input_R3            "/1 -> Mux/3
  "Mot_Input_L1            "/1 -> Mux/4
  "Mot_Input_L2            "/1 -> Mux/5
  "Mot_Input_L3            "/1 -> Mux/6
  "Torque_RW1_RH@Arm1      "/1 -> Mux/7
  "Torque_RW1_LH@Arm1      "/1 -> Mux/8
  "DamperOFF_RW1_RH@Arm1   "/1 -> Mux/9
  "DamperOFF_RW1_LH@Arm1   "/1 -> Mux/10
  StaticTorque_RW1_RH@Arm1/1 -> Mux/11
  StaticTorque_RW1_LH@Arm1/1 -> Mux/12
  "SpringOFF_RW1_RH@Arm1   "/1 -> Mux/13
  "SpringOFF_RW1_LH@Arm1   "/1 -> Mux/14
  "Torque_RW2_RH@Arm2      "/1 -> Mux/15
  "Torque_RW2_LH@Arm2      "/1 -> Mux/16
  "DamperOFF_RW2_RH@Arm2   "/1 -> Mux/17
  "DamperOFF_RW2_LH@Arm2   "/1 -> Mux/18
  StaticTorque_RW2_RH@Arm2/1 -> Mux/19
  StaticTorque_RW2_LH@Arm2/1 -> Mux/20
  "SpringOFF_RW2_RH@Arm2   "/1 -> Mux/21
  "SpringOFF_RW2_LH@Arm2   "/1 -> Mux/22

== system control_cdr_hybrid/Vehicle Velocity Controller (Driver Model)/L1_controller ==
  Ref_Vel : Inport
  Feedback_Vel : Inport  Port=2
  Subsystem : Subsystem
      mask Display: disp('PI');
  Sum : Sum  Inputs=|+-  SaturateOnIntegerOverflow=on  InputSameDT=on  OutDataTypeStr=Inherit: Same as first input
  Torque_L1 : Outport
  wires:
  Sum/1 -> Subsystem/1(In1)
  Subsystem/1(Out1) -> Torque_L1/1
  Ref_Vel/1 -> Sum/1
  Feedback_Vel/1 -> Sum/2

== system control_cdr_hybrid/Vehicle Velocity Controller (Driver Model)/R1_controller ==
  Ref_Vel : Inport
  Feedback_Vel : Inport  Port=2
  Subsystem : Subsystem
      mask Display: disp('PI');
  Sum : Sum  Inputs=|+-  SaturateOnIntegerOverflow=on  InputSameDT=on  OutDataTypeStr=Inherit: Same as first input
  Torque_R1 : Outport
  wires:
  Feedback_Vel/1 -> Sum/2
  Ref_Vel/1 -> Sum/1
  Subsystem/1(Out1) -> Torque_R1/1
  Sum/1 -> Subsystem/1(In1)

== system control_cdr_hybrid/Vehicle Velocity Controller (Driver Model)/R2_controller ==
  Ref_Vel : Inport
  Feedback_Vel : Inport  Port=2
  Subsystem : Subsystem
      mask Display: disp('PI');
  Sum : Sum  Inputs=|+-  SaturateOnIntegerOverflow=on  InputSameDT=on  OutDataTypeStr=Inherit: Same as first input
  Torque_R2 : Outport
  wires:
  Sum/1 -> Subsystem/1(In1)
  Subsystem/1(Out1) -> Torque_R2/1
  Ref_Vel/1 -> Sum/1
  Feedback_Vel/1 -> Sum/2

== system control_cdr_hybrid/Vehicle Velocity Controller (Driver Model)/R3_controller ==
  Ref_Vel : Inport
  Feedback_Vel : Inport  Port=2
  Subsystem : Subsystem
      mask Display: disp('PI');
  Sum : Sum  Inputs=|+-  SaturateOnIntegerOverflow=on  InputSameDT=on  OutDataTypeStr=Inherit: Same as first input
  Torque_R3 : Outport
  wires:
  Feedback_Vel/1 -> Sum/2
  Ref_Vel/1 -> Sum/1
  Subsystem/1(Out1) -> Torque_R3/1
  Sum/1 -> Subsystem/1(In1)

== system control_cdr_hybrid/Vehicle Velocity Controller (Driver Model)/normal case velocity control profile ==
  Demux : Demux  Tag=STV Demux  Outputs=1
  FromWs : FromWorkspace  Tag=STV FromWs  VariableName=tuvar  SampleTime=0.001  OutputAfterFinalValue=Holding final value  SigBuilderData=DataTag0  VnvData=DataTag1
      SigBuilderData=|
      | common.afterFinalStr = 'Hold final value'
      | common.sampleTime = '0.001'
      | dataSet.timeRange = [0 100]
      | dataSet.name = 'Group 1'
      | sbobj.Groups.Name = 'Group 1'
      | sbobj.Groups.Signals.Name = 'Signal 1'
      | sbobj.Groups.Signals.XData = [0 25 45 100]
      | sbobj.Groups.Signals.YData = [0 0 1 1]
  Signal 1 : Outport  Tag=STV Outport
  wires:
  Demux/1 -> Signal 1/1
  FromWs/1 -> Demux/1

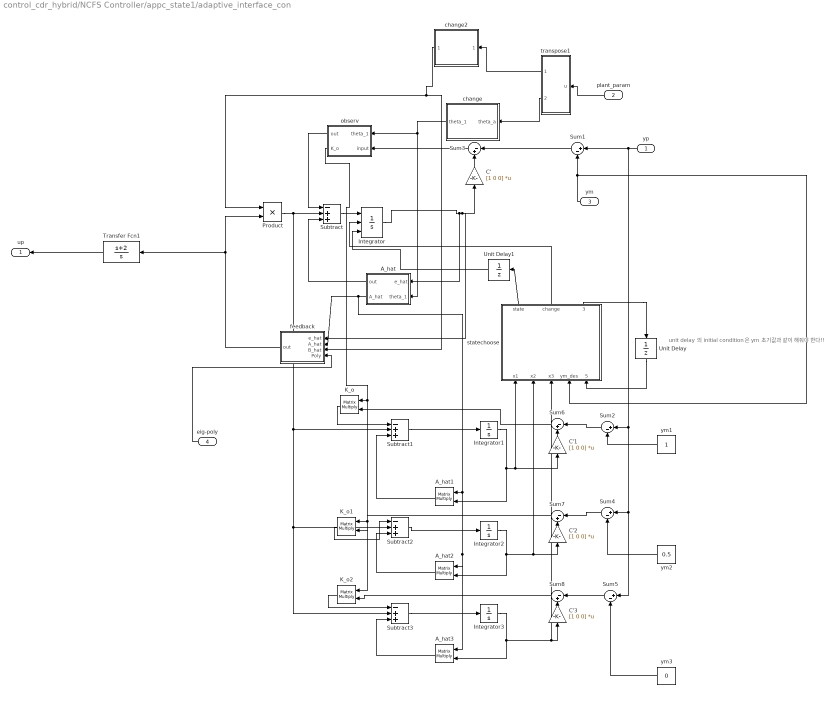
== system control_cdr_hybrid/NCFS Controller/appc_state1/adaptive_interface_con ==
  note: unit delay 의 initial condition은 ym 초기값과 같이 해줘야 한다!!
  yp : Inport
  plant_param : Inport  Port=2
  ym : Inport  Port=3
  eig-poly : Inport  Port=4
  A_hat : MATLAB Function  TreatAsAtomicUnit=on
  A_hat1 : Product  Multiplication=Matrix(*)  RndMeth=Zero
  A_hat2 : Product  Multiplication=Matrix(*)  RndMeth=Zero
  A_hat3 : Product  Multiplication=Matrix(*)  RndMeth=Zero
  C'{,1..3} (4 alike) : Gain  Gain=[1 0 0]  Multiplication=Matrix(K*u)
  Integrator : Integrator  ExternalReset=level  InitialConditionSource=external
  Integrator1 : Integrator
  Integrator2 : Integrator
  Integrator3 : Integrator
  K_o : Product  Multiplication=Matrix(*)  RndMeth=Zero
  K_o1 : Product  Multiplication=Matrix(*)  RndMeth=Zero
  K_o2 : Product  Multiplication=Matrix(*)  RndMeth=Zero
  Product : Product  RndMeth=Zero
  Subtract{,1..3} (4 alike) : Sum  Inputs=-++
  Sum{1..2,4..5} (4 alike) : Sum  Inputs=|+-
  Sum{3,6..8} (4 alike) : Sum  Inputs=|-+
  Transfer Fcn1 : TransferFcn  Numerator=[1 2]  Denominator=[1 0]
  Unit Delay : UnitDelay  X0=0.8  SampleTime=-1
  Unit Delay1 : UnitDelay  X0=0.8  SampleTime=-1
  change : MATLAB Function  TreatAsAtomicUnit=on
  change2 : MATLAB Function  TreatAsAtomicUnit=on
  feedback : MATLAB Function  TreatAsAtomicUnit=on
  observ : MATLAB Function  TreatAsAtomicUnit=on
  statechoose : MATLAB Function  TreatAsAtomicUnit=on
  transpose1 : MATLAB Function  TreatAsAtomicUnit=on
  ym1 : Constant
  ym2 : Constant  Value=0.5
  ym3 : Constant  Value=0
  up : Outport
  wires:
  Subtract/1 -> Integrator/1
  transpose1/2(theta_a) -> change/1(theta_a)
  A_hat/1(out) -> Subtract/3
  transpose1/1(theta_b) -> change2/1(theta_b)
  Product/1 -> Subtract/2, Subtract1/2, Subtract2/2, Subtract3/2
  A_hat/2(A_hat) -> feedback/2(A_hat), A_hat2/1, A_hat3/1, A_hat1/1
  feedback/1(out) -> Product/2, Transfer Fcn1/1
  C'/1 -> Sum3/2
  Sum3/1 -> observ/2(input)
  observ/1(out) -> Subtract/1
  change/1(theta_1) -> A_hat/2(theta_1), observ/1(theta_1)
  change2/1(theta_2) -> feedback/3(B_hat), Product/1
  Transfer Fcn1/1 -> up/1
  plant_param/1 -> transpose1/1(u)
  yp/1 -> Sum1/1, Sum2/1, Sum4/1, Sum5/1
  ym/1 -> Sum1/2, statechoose/4(ym_des)
  Sum1/1 -> Sum3/1
  ym2/1 -> Sum4/2
  ym1/1 -> Sum2/2
  ym3/1 -> Sum5/2
  Subtract1/1 -> Integrator1/1
  Integrator1/1 -> statechoose/1(x1), C'1/1, A_hat1/2
  Subtract2/1 -> Integrator2/1
  Subtract3/1 -> Integrator3/1
  Integrator2/1 -> A_hat2/2, C'2/1, statechoose/2(x2)
  Integrator3/1 -> A_hat3/2, C'3/1, statechoose/3(x3)
  Sum2/1 -> Sum6/1
  C'1/1 -> Sum6/2
  Sum4/1 -> Sum7/1
  C'2/1 -> Sum7/2
  Sum5/1 -> Sum8/1
  C'3/1 -> Sum8/2
  A_hat3/1 -> Subtract3/3
  A_hat2/1 -> Subtract2/3
  A_hat1/1 -> Subtract1/3
  observ/2(K_o) -> K_o/1, K_o1/1, K_o2/1
  Sum6/1 -> K_o/2
  Sum7/1 -> K_o1/2
  Sum8/1 -> K_o2/2
  K_o/1 -> Subtract1/1
  K_o1/1 -> Subtract2/1
  K_o2/1 -> Subtract3/1
  statechoose/3(ym_des_mem) -> Unit Delay/1
  Unit Delay/1 -> statechoose/5(ym_des_before)
  Integrator/1 -> A_hat/1(e_hat), feedback/1(e_hat), C'/1
  statechoose/2(change) -> Integrator/2
  statechoose/1(state) -> Unit Delay1/1
  Unit Delay1/1 -> Integrator/3
  eig-poly/1 -> feedback/4(Poly)

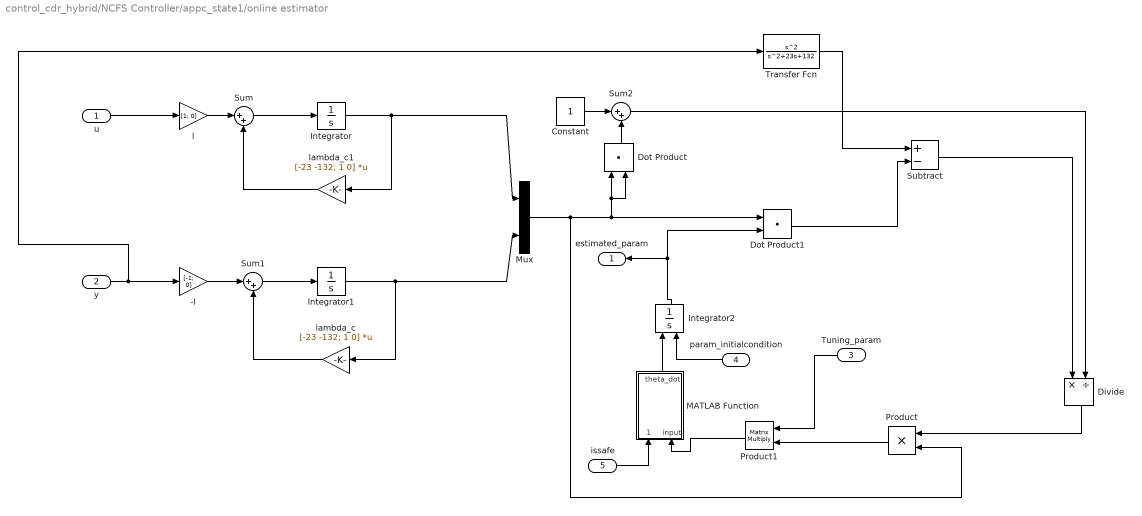
== system control_cdr_hybrid/NCFS Controller/appc_state1/online estimator ==
  u : Inport
  y : Inport  Port=2
  Tuning_param : Inport  Port=3
  param_initialcondition : Inport  Port=4
  issafe : Inport  Port=5
  -l : Gain  Gain=[-1; 0]
  Constant : Constant
  Divide : Product  Inputs=*/
  Dot Product : DotProduct  InputSameDT=on  OutDataTypeStr=Inherit: Inherit via internal rule
  Dot Product1 : DotProduct  InputSameDT=on  OutDataTypeStr=Inherit: Inherit via internal rule
  Integrator : Integrator
  Integrator1 : Integrator
  Integrator2 : Integrator  InitialConditionSource=external  InitialCondition=[1; 2; 4; 3]
  MATLAB Function : MATLAB Function  TreatAsAtomicUnit=on
  Mux : Mux  Inputs=2
  Product : Product  RndMeth=Zero
  Product1 : Product  Multiplication=Matrix(*)  RndMeth=Zero
  Subtract : Sum  Inputs=+-
  Sum : Sum  Inputs=|++
  Sum1 : Sum  Inputs=|++
  Sum2 : Sum  Inputs=|++
  Transfer Fcn : TransferFcn  Numerator=[1 0 0]  Denominator=[1 23 132]
  l : Gain  Gain=[1; 0]
  lambda_c : Gain  Gain=[-23 -132; 1 0]  Multiplication=Matrix(K*u)
  lambda_c1 : Gain  Gain=[-23 -132; 1 0]  Multiplication=Matrix(K*u)
  estimated_param : Outport
  wires:
  y/1 -> -l/1, Transfer Fcn/1
  u/1 -> l/1
  -l/1 -> Sum1/1
  l/1 -> Sum/1
  Sum/1 -> Integrator/1
  Integrator1/1 -> lambda_c/1, Mux/2
  Integrator/1 -> lambda_c1/1, Mux/1
  lambda_c1/1 -> Sum/2
  lambda_c/1 -> Sum1/2
  Mux/1 -> Dot Product/1, Dot Product/2, Dot Product1/1, Product/2
  Constant/1 -> Sum2/1
  Dot Product/1 -> Sum2/2
  Transfer Fcn/1 -> Subtract/1
  Dot Product1/1 -> Subtract/2
  Subtract/1 -> Divide/1
  Sum2/1 -> Divide/2
  Divide/1 -> Product/1
  Integrator2/1 -> Dot Product1/2, estimated_param/1
  Sum1/1 -> Integrator1/1
  Tuning_param/1 -> Product1/1
  Product/1 -> Product1/2
  param_initialcondition/1 -> Integrator2/2
  MATLAB Function/1(theta_dot) -> Integrator2/1
  issafe/1 -> MATLAB Function/1(issafe)
  Product1/1 -> MATLAB Function/2(input)

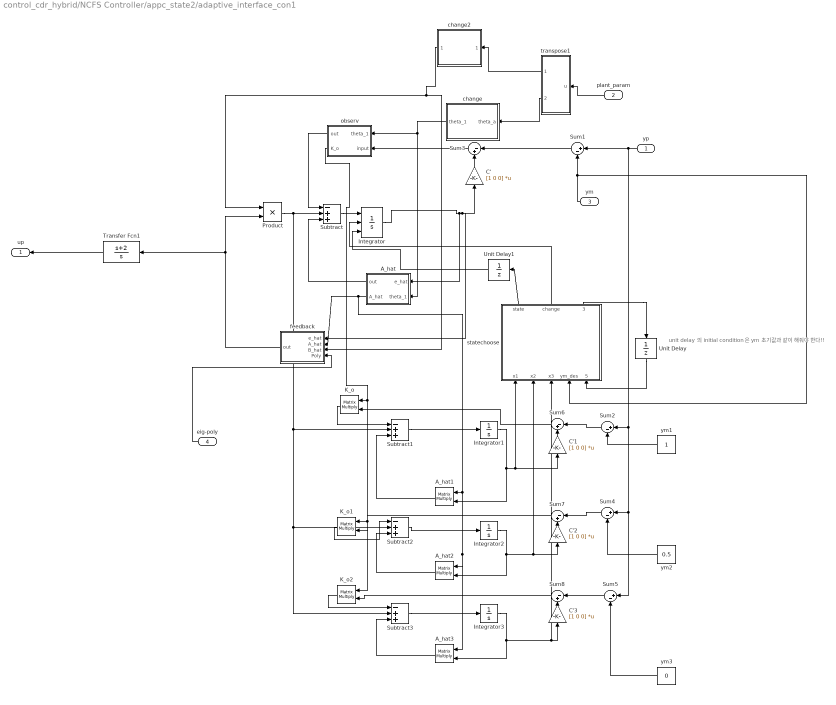
== system control_cdr_hybrid/NCFS Controller/appc_state2/adaptive_interface_con1 ==
  note: unit delay 의 initial condition은 ym 초기값과 같이 해줘야 한다!!
  yp : Inport
  plant_param : Inport  Port=2
  ym : Inport  Port=3
  eig-poly : Inport  Port=4
  A_hat : MATLAB Function  TreatAsAtomicUnit=on
  A_hat1 : Product  Multiplication=Matrix(*)  RndMeth=Zero
  A_hat2 : Product  Multiplication=Matrix(*)  RndMeth=Zero
  A_hat3 : Product  Multiplication=Matrix(*)  RndMeth=Zero
  C'{,1..3} (4 alike) : Gain  Gain=[1 0 0]  Multiplication=Matrix(K*u)
  Integrator : Integrator  ExternalReset=level  InitialConditionSource=external
  Integrator1 : Integrator
  Integrator2 : Integrator
  Integrator3 : Integrator
  K_o : Product  Multiplication=Matrix(*)  RndMeth=Zero
  K_o1 : Product  Multiplication=Matrix(*)  RndMeth=Zero
  K_o2 : Product  Multiplication=Matrix(*)  RndMeth=Zero
  Product : Product  RndMeth=Zero
  Subtract{,1..3} (4 alike) : Sum  Inputs=-++
  Sum{1..2,4..5} (4 alike) : Sum  Inputs=|+-
  Sum{3,6..8} (4 alike) : Sum  Inputs=|-+
  Transfer Fcn1 : TransferFcn  Numerator=[1 2]  Denominator=[1 0]
  Unit Delay : UnitDelay  X0=0.8  SampleTime=-1
  Unit Delay1 : UnitDelay  X0=0.8  SampleTime=-1
  change : MATLAB Function  TreatAsAtomicUnit=on
  change2 : MATLAB Function  TreatAsAtomicUnit=on
  feedback : MATLAB Function  TreatAsAtomicUnit=on
  observ : MATLAB Function  TreatAsAtomicUnit=on
  statechoose : MATLAB Function  TreatAsAtomicUnit=on
  transpose1 : MATLAB Function  TreatAsAtomicUnit=on
  ym1 : Constant
  ym2 : Constant  Value=0.5
  ym3 : Constant  Value=0
  up : Outport
  wires:
  Subtract/1 -> Integrator/1
  transpose1/2(theta_a) -> change/1(theta_a)
  A_hat/1(out) -> Subtract/3
  transpose1/1(theta_b) -> change2/1(theta_b)
  Product/1 -> Subtract/2, Subtract1/2, Subtract2/2, Subtract3/2
  A_hat/2(A_hat) -> feedback/2(A_hat), A_hat1/1, A_hat2/1, A_hat3/1
  feedback/1(out) -> Product/2, Transfer Fcn1/1
  C'/1 -> Sum3/2
  Sum3/1 -> observ/2(input)
  observ/1(out) -> Subtract/1
  change/1(theta_1) -> A_hat/2(theta_1), observ/1(theta_1)
  change2/1(theta_2) -> feedback/3(B_hat), Product/1
  Transfer Fcn1/1 -> up/1
  plant_param/1 -> transpose1/1(u)
  yp/1 -> Sum1/1, Sum2/1, Sum4/1, Sum5/1
  ym/1 -> Sum1/2, statechoose/4(ym_des)
  Sum1/1 -> Sum3/1
  ym2/1 -> Sum4/2
  ym1/1 -> Sum2/2
  ym3/1 -> Sum5/2
  Subtract1/1 -> Integrator1/1
  Integrator1/1 -> A_hat1/2, statechoose/1(x1), C'1/1
  Subtract2/1 -> Integrator2/1
  Subtract3/1 -> Integrator3/1
  Integrator2/1 -> A_hat2/2, C'2/1, statechoose/2(x2)
  Integrator3/1 -> A_hat3/2, C'3/1, statechoose/3(x3)
  Sum2/1 -> Sum6/1
  C'1/1 -> Sum6/2
  Sum4/1 -> Sum7/1
  C'2/1 -> Sum7/2
  Sum5/1 -> Sum8/1
  C'3/1 -> Sum8/2
  A_hat3/1 -> Subtract3/3
  A_hat2/1 -> Subtract2/3
  A_hat1/1 -> Subtract1/3
  observ/2(K_o) -> K_o/1, K_o1/1, K_o2/1
  Sum6/1 -> K_o/2
  Sum7/1 -> K_o1/2
  Sum8/1 -> K_o2/2
  K_o/1 -> Subtract1/1
  K_o1/1 -> Subtract2/1
  K_o2/1 -> Subtract3/1
  statechoose/3(ym_des_mem) -> Unit Delay/1
  Unit Delay/1 -> statechoose/5(ym_des_before)
  Integrator/1 -> A_hat/1(e_hat), feedback/1(e_hat), C'/1
  statechoose/2(change) -> Integrator/2
  statechoose/1(state) -> Unit Delay1/1
  Unit Delay1/1 -> Integrator/3
  eig-poly/1 -> feedback/4(Poly)

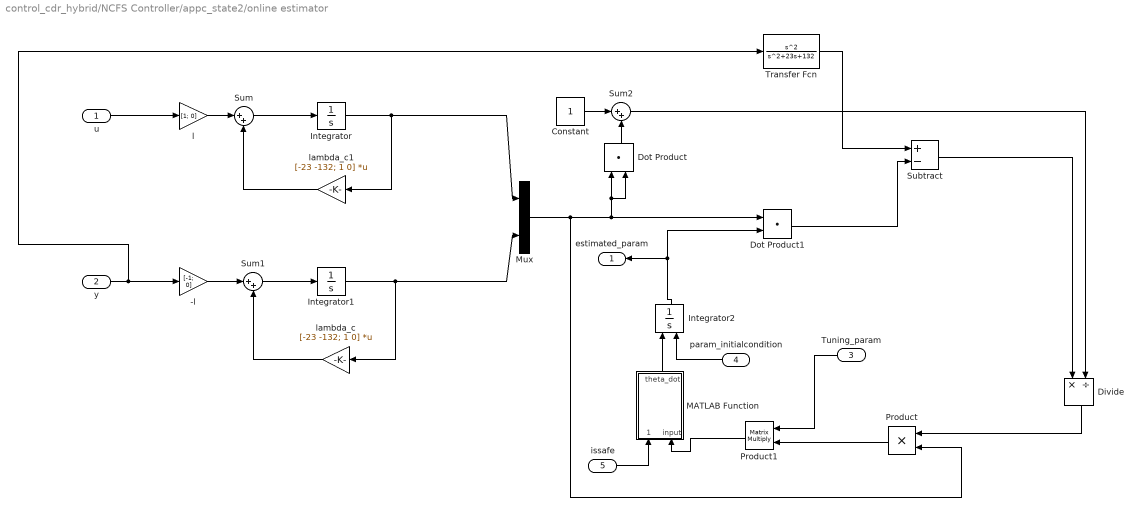
== system control_cdr_hybrid/NCFS Controller/appc_state2/online estimator ==
  u : Inport
  y : Inport  Port=2
  Tuning_param : Inport  Port=3
  param_initialcondition : Inport  Port=4
  issafe : Inport  Port=5
  -l : Gain  Gain=[-1; 0]
  Constant : Constant
  Divide : Product  Inputs=*/
  Dot Product : DotProduct  InputSameDT=on  OutDataTypeStr=Inherit: Inherit via internal rule
  Dot Product1 : DotProduct  InputSameDT=on  OutDataTypeStr=Inherit: Inherit via internal rule
  Integrator : Integrator
  Integrator1 : Integrator
  Integrator2 : Integrator  InitialConditionSource=external  InitialCondition=[1; 2; 4; 3]
  MATLAB Function : MATLAB Function  TreatAsAtomicUnit=on
  Mux : Mux  Inputs=2
  Product : Product  RndMeth=Zero
  Product1 : Product  Multiplication=Matrix(*)  RndMeth=Zero
  Subtract : Sum  Inputs=+-
  Sum : Sum  Inputs=|++
  Sum1 : Sum  Inputs=|++
  Sum2 : Sum  Inputs=|++
  Transfer Fcn : TransferFcn  Numerator=[1 0 0]  Denominator=[1 23 132]
  l : Gain  Gain=[1; 0]
  lambda_c : Gain  Gain=[-23 -132; 1 0]  Multiplication=Matrix(K*u)
  lambda_c1 : Gain  Gain=[-23 -132; 1 0]  Multiplication=Matrix(K*u)
  estimated_param : Outport
  wires:
  y/1 -> -l/1, Transfer Fcn/1
  u/1 -> l/1
  -l/1 -> Sum1/1
  l/1 -> Sum/1
  Sum/1 -> Integrator/1
  Integrator1/1 -> lambda_c/1, Mux/2
  Integrator/1 -> lambda_c1/1, Mux/1
  lambda_c1/1 -> Sum/2
  lambda_c/1 -> Sum1/2
  Mux/1 -> Dot Product/1, Dot Product/2, Dot Product1/1, Product/2
  Constant/1 -> Sum2/1
  Dot Product/1 -> Sum2/2
  Transfer Fcn/1 -> Subtract/1
  Dot Product1/1 -> Subtract/2
  Subtract/1 -> Divide/1
  Sum2/1 -> Divide/2
  Divide/1 -> Product/1
  Integrator2/1 -> Dot Product1/2, estimated_param/1
  Sum1/1 -> Integrator1/1
  Tuning_param/1 -> Product1/1
  Product/1 -> Product1/2
  param_initialcondition/1 -> Integrator2/2
  MATLAB Function/1(theta_dot) -> Integrator2/1
  issafe/1 -> MATLAB Function/1(issafe)
  Product1/1 -> MATLAB Function/2(input)

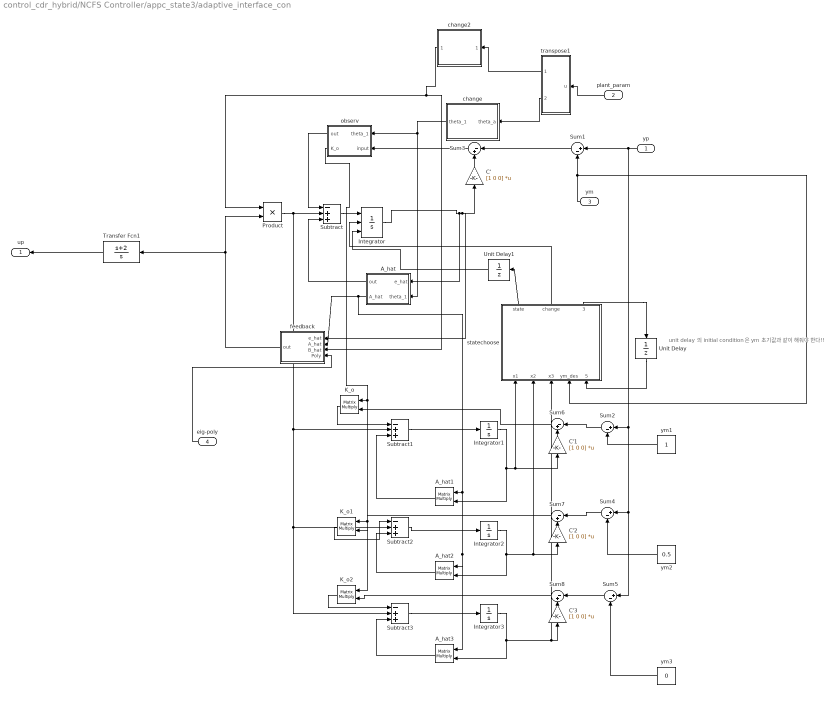
== system control_cdr_hybrid/NCFS Controller/appc_state3/adaptive_interface_con ==
  note: unit delay 의 initial condition은 ym 초기값과 같이 해줘야 한다!!
  yp : Inport
  plant_param : Inport  Port=2
  ym : Inport  Port=3
  eig-poly : Inport  Port=4
  A_hat : MATLAB Function  TreatAsAtomicUnit=on
  A_hat1 : Product  Multiplication=Matrix(*)  RndMeth=Zero
  A_hat2 : Product  Multiplication=Matrix(*)  RndMeth=Zero
  A_hat3 : Product  Multiplication=Matrix(*)  RndMeth=Zero
  C'{,1..3} (4 alike) : Gain  Gain=[1 0 0]  Multiplication=Matrix(K*u)
  Integrator : Integrator  ExternalReset=level  InitialConditionSource=external
  Integrator1 : Integrator
  Integrator2 : Integrator
  Integrator3 : Integrator
  K_o : Product  Multiplication=Matrix(*)  RndMeth=Zero
  K_o1 : Product  Multiplication=Matrix(*)  RndMeth=Zero
  K_o2 : Product  Multiplication=Matrix(*)  RndMeth=Zero
  Product : Product  RndMeth=Zero
  Subtract{,1..3} (4 alike) : Sum  Inputs=-++
  Sum{1..2,4..5} (4 alike) : Sum  Inputs=|+-
  Sum{3,6..8} (4 alike) : Sum  Inputs=|-+
  Transfer Fcn1 : TransferFcn  Numerator=[1 2]  Denominator=[1 0]
  Unit Delay : UnitDelay  X0=0.8  SampleTime=-1
  Unit Delay1 : UnitDelay  X0=0.8  SampleTime=-1
  change : MATLAB Function  TreatAsAtomicUnit=on
  change2 : MATLAB Function  TreatAsAtomicUnit=on
  feedback : MATLAB Function  TreatAsAtomicUnit=on
  observ : MATLAB Function  TreatAsAtomicUnit=on
  statechoose : MATLAB Function  TreatAsAtomicUnit=on
  transpose1 : MATLAB Function  TreatAsAtomicUnit=on
  ym1 : Constant
  ym2 : Constant  Value=0.5
  ym3 : Constant  Value=0
  up : Outport
  wires:
  Subtract/1 -> Integrator/1
  transpose1/2(theta_a) -> change/1(theta_a)
  A_hat/1(out) -> Subtract/3
  transpose1/1(theta_b) -> change2/1(theta_b)
  Product/1 -> Subtract/2, Subtract1/2, Subtract2/2, Subtract3/2
  A_hat/2(A_hat) -> feedback/2(A_hat), A_hat1/1, A_hat2/1, A_hat3/1
  feedback/1(out) -> Product/2, Transfer Fcn1/1
  C'/1 -> Sum3/2
  Sum3/1 -> observ/2(input)
  observ/1(out) -> Subtract/1
  change/1(theta_1) -> A_hat/2(theta_1), observ/1(theta_1)
  change2/1(theta_2) -> feedback/3(B_hat), Product/1
  Transfer Fcn1/1 -> up/1
  plant_param/1 -> transpose1/1(u)
  yp/1 -> Sum1/1, Sum2/1, Sum4/1, Sum5/1
  ym/1 -> Sum1/2, statechoose/4(ym_des)
  Sum1/1 -> Sum3/1
  ym2/1 -> Sum4/2
  ym1/1 -> Sum2/2
  ym3/1 -> Sum5/2
  Subtract1/1 -> Integrator1/1
  Integrator1/1 -> A_hat1/2, statechoose/1(x1), C'1/1
  Subtract2/1 -> Integrator2/1
  Subtract3/1 -> Integrator3/1
  Integrator2/1 -> A_hat2/2, C'2/1, statechoose/2(x2)
  Integrator3/1 -> A_hat3/2, C'3/1, statechoose/3(x3)
  Sum2/1 -> Sum6/1
  C'1/1 -> Sum6/2
  Sum4/1 -> Sum7/1
  C'2/1 -> Sum7/2
  Sum5/1 -> Sum8/1
  C'3/1 -> Sum8/2
  A_hat3/1 -> Subtract3/3
  A_hat2/1 -> Subtract2/3
  A_hat1/1 -> Subtract1/3
  observ/2(K_o) -> K_o/1, K_o1/1, K_o2/1
  Sum6/1 -> K_o/2
  Sum7/1 -> K_o1/2
  Sum8/1 -> K_o2/2
  K_o/1 -> Subtract1/1
  K_o1/1 -> Subtract2/1
  K_o2/1 -> Subtract3/1
  statechoose/3(ym_des_mem) -> Unit Delay/1
  Unit Delay/1 -> statechoose/5(ym_des_before)
  Integrator/1 -> A_hat/1(e_hat), feedback/1(e_hat), C'/1
  statechoose/2(change) -> Integrator/2
  statechoose/1(state) -> Unit Delay1/1
  Unit Delay1/1 -> Integrator/3
  eig-poly/1 -> feedback/4(Poly)

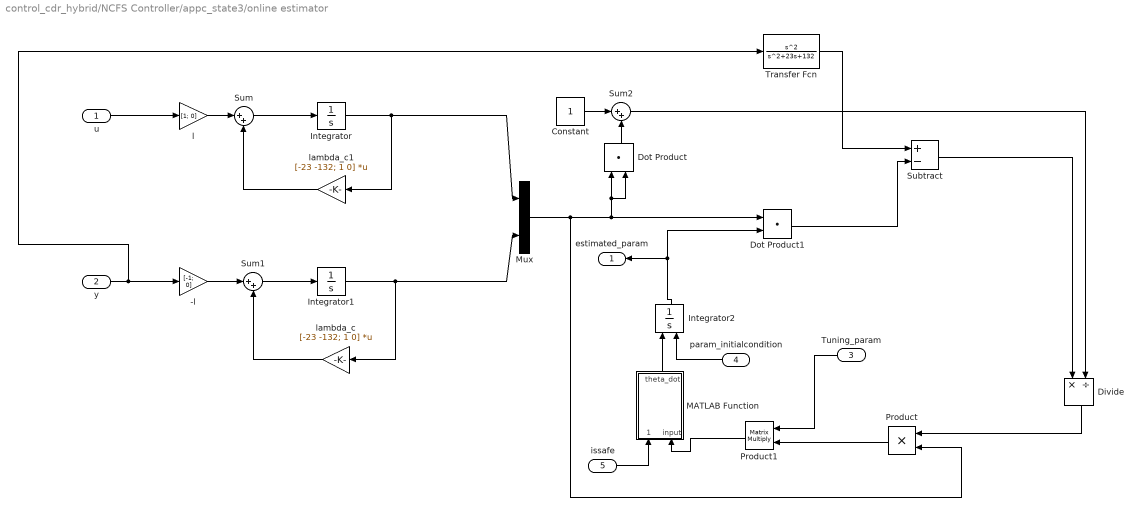
== system control_cdr_hybrid/NCFS Controller/appc_state3/online estimator ==
  u : Inport
  y : Inport  Port=2
  Tuning_param : Inport  Port=3
  param_initialcondition : Inport  Port=4
  issafe : Inport  Port=5
  -l : Gain  Gain=[-1; 0]
  Constant : Constant
  Divide : Product  Inputs=*/
  Dot Product : DotProduct  InputSameDT=on  OutDataTypeStr=Inherit: Inherit via internal rule
  Dot Product1 : DotProduct  InputSameDT=on  OutDataTypeStr=Inherit: Inherit via internal rule
  Integrator : Integrator
  Integrator1 : Integrator
  Integrator2 : Integrator  InitialConditionSource=external  InitialCondition=[1; 2; 4; 3]
  MATLAB Function : MATLAB Function  TreatAsAtomicUnit=on
  Mux : Mux  Inputs=2
  Product : Product  RndMeth=Zero
  Product1 : Product  Multiplication=Matrix(*)  RndMeth=Zero
  Subtract : Sum  Inputs=+-
  Sum : Sum  Inputs=|++
  Sum1 : Sum  Inputs=|++
  Sum2 : Sum  Inputs=|++
  Transfer Fcn : TransferFcn  Numerator=[1 0 0]  Denominator=[1 23 132]
  l : Gain  Gain=[1; 0]
  lambda_c : Gain  Gain=[-23 -132; 1 0]  Multiplication=Matrix(K*u)
  lambda_c1 : Gain  Gain=[-23 -132; 1 0]  Multiplication=Matrix(K*u)
  estimated_param : Outport
  wires:
  y/1 -> -l/1, Transfer Fcn/1
  u/1 -> l/1
  -l/1 -> Sum1/1
  l/1 -> Sum/1
  Sum/1 -> Integrator/1
  Integrator1/1 -> lambda_c/1, Mux/2
  Integrator/1 -> lambda_c1/1, Mux/1
  lambda_c1/1 -> Sum/2
  lambda_c/1 -> Sum1/2
  Mux/1 -> Dot Product/1, Dot Product/2, Dot Product1/1, Product/2
  Constant/1 -> Sum2/1
  Dot Product/1 -> Sum2/2
  Transfer Fcn/1 -> Subtract/1
  Dot Product1/1 -> Subtract/2
  Subtract/1 -> Divide/1
  Sum2/1 -> Divide/2
  Divide/1 -> Product/1
  Integrator2/1 -> Dot Product1/2, estimated_param/1
  Sum1/1 -> Integrator1/1
  Tuning_param/1 -> Product1/1
  Product/1 -> Product1/2
  param_initialcondition/1 -> Integrator2/2
  MATLAB Function/1(theta_dot) -> Integrator2/1
  issafe/1 -> MATLAB Function/1(issafe)
  Product1/1 -> MATLAB Function/2(input)

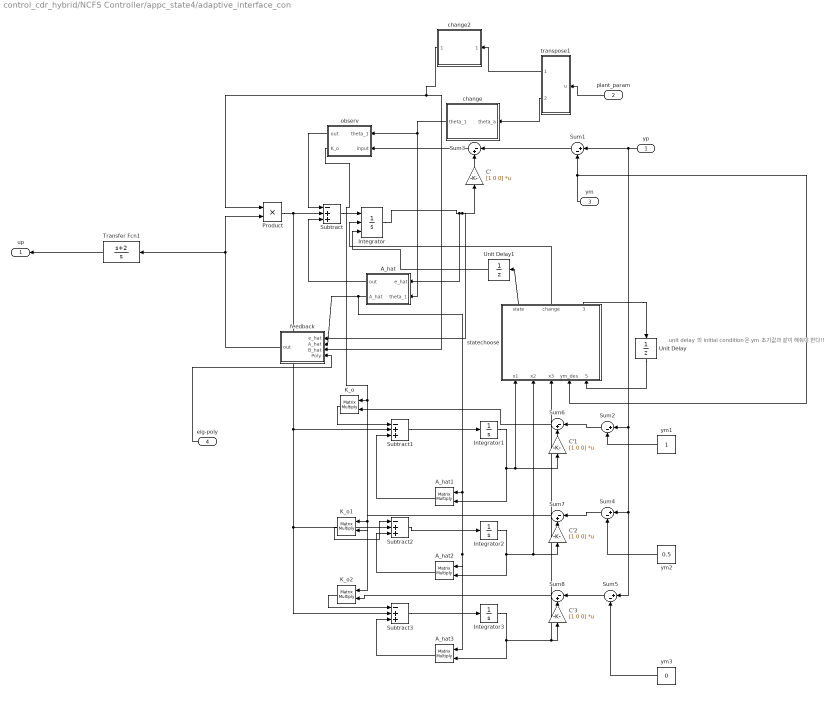
== system control_cdr_hybrid/NCFS Controller/appc_state4/adaptive_interface_con ==
  note: unit delay 의 initial condition은 ym 초기값과 같이 해줘야 한다!!
  yp : Inport
  plant_param : Inport  Port=2
  ym : Inport  Port=3
  eig-poly : Inport  Port=4
  A_hat : MATLAB Function  TreatAsAtomicUnit=on
  A_hat1 : Product  Multiplication=Matrix(*)  RndMeth=Zero
  A_hat2 : Product  Multiplication=Matrix(*)  RndMeth=Zero
  A_hat3 : Product  Multiplication=Matrix(*)  RndMeth=Zero
  C'{,1..3} (4 alike) : Gain  Gain=[1 0 0]  Multiplication=Matrix(K*u)
  Integrator : Integrator  ExternalReset=level  InitialConditionSource=external
  Integrator1 : Integrator
  Integrator2 : Integrator
  Integrator3 : Integrator
  K_o : Product  Multiplication=Matrix(*)  RndMeth=Zero
  K_o1 : Product  Multiplication=Matrix(*)  RndMeth=Zero
  K_o2 : Product  Multiplication=Matrix(*)  RndMeth=Zero
  Product : Product  RndMeth=Zero
  Subtract{,1..3} (4 alike) : Sum  Inputs=-++
  Sum{1..2,4..5} (4 alike) : Sum  Inputs=|+-
  Sum{3,6..8} (4 alike) : Sum  Inputs=|-+
  Transfer Fcn1 : TransferFcn  Numerator=[1 2]  Denominator=[1 0]
  Unit Delay : UnitDelay  X0=0.8  SampleTime=-1
  Unit Delay1 : UnitDelay  X0=0.8  SampleTime=-1
  change : MATLAB Function  TreatAsAtomicUnit=on
  change2 : MATLAB Function  TreatAsAtomicUnit=on
  feedback : MATLAB Function  TreatAsAtomicUnit=on
  observ : MATLAB Function  TreatAsAtomicUnit=on
  statechoose : MATLAB Function  TreatAsAtomicUnit=on
  transpose1 : MATLAB Function  TreatAsAtomicUnit=on
  ym1 : Constant
  ym2 : Constant  Value=0.5
  ym3 : Constant  Value=0
  up : Outport
  wires:
  Subtract/1 -> Integrator/1
  transpose1/2(theta_a) -> change/1(theta_a)
  A_hat/1(out) -> Subtract/3
  transpose1/1(theta_b) -> change2/1(theta_b)
  Product/1 -> Subtract/2, Subtract1/2, Subtract2/2, Subtract3/2
  A_hat/2(A_hat) -> feedback/2(A_hat), A_hat1/1, A_hat2/1, A_hat3/1
  feedback/1(out) -> Product/2, Transfer Fcn1/1
  C'/1 -> Sum3/2
  Sum3/1 -> observ/2(input)
  observ/1(out) -> Subtract/1
  change/1(theta_1) -> A_hat/2(theta_1), observ/1(theta_1)
  change2/1(theta_2) -> feedback/3(B_hat), Product/1
  Transfer Fcn1/1 -> up/1
  plant_param/1 -> transpose1/1(u)
  yp/1 -> Sum1/1, Sum2/1, Sum4/1, Sum5/1
  ym/1 -> Sum1/2, statechoose/4(ym_des)
  Sum1/1 -> Sum3/1
  ym2/1 -> Sum4/2
  ym1/1 -> Sum2/2
  ym3/1 -> Sum5/2
  Subtract1/1 -> Integrator1/1
  Integrator1/1 -> A_hat1/2, statechoose/1(x1), C'1/1
  Subtract2/1 -> Integrator2/1
  Subtract3/1 -> Integrator3/1
  Integrator2/1 -> A_hat2/2, C'2/1, statechoose/2(x2)
  Integrator3/1 -> A_hat3/2, C'3/1, statechoose/3(x3)
  Sum2/1 -> Sum6/1
  C'1/1 -> Sum6/2
  Sum4/1 -> Sum7/1
  C'2/1 -> Sum7/2
  Sum5/1 -> Sum8/1
  C'3/1 -> Sum8/2
  A_hat3/1 -> Subtract3/3
  A_hat2/1 -> Subtract2/3
  A_hat1/1 -> Subtract1/3
  observ/2(K_o) -> K_o/1, K_o1/1, K_o2/1
  Sum6/1 -> K_o/2
  Sum7/1 -> K_o1/2
  Sum8/1 -> K_o2/2
  K_o/1 -> Subtract1/1
  K_o1/1 -> Subtract2/1
  K_o2/1 -> Subtract3/1
  statechoose/3(ym_des_mem) -> Unit Delay/1
  Unit Delay/1 -> statechoose/5(ym_des_before)
  Integrator/1 -> A_hat/1(e_hat), feedback/1(e_hat), C'/1
  statechoose/2(change) -> Integrator/2
  statechoose/1(state) -> Unit Delay1/1
  Unit Delay1/1 -> Integrator/3
  eig-poly/1 -> feedback/4(Poly)
